simulink library "SimpleTrackedSurveillanceBlock"  (R2018b)
settings: Solver=VariableStepAuto  StartTime=0.0  StopTime=10.0  RelTol=1e-3
undefined symbols (not defined in the file): ac1_ac2_deVar_ft2ps2, ac1_ac2_dhVar_ft2ps2, ac1_ac2_dnVar_ft2ps2, ac1_ac2_east_position_error_ft, ac1_ac2_east_velocity_error_fps, ac1_ac2_eVar_ft2, ac1_ac2_horizontal_position_jitter_stddev_ft, ac1_ac2_horizontal_velocity_jitter_stddev_fps, ac1_ac2_hVar_ft2, ac1_ac2_north_position_error_ft, ac1_ac2_north_velocity_error_fps, ac1_ac2_nVar_ft2, ac1_ac2_seed1, ac1_ac2_seed2, ac1_ac2_seed3, ac1_ac2_seed4, ac1_ac2_seed5, ac1_ac2_seed6, ac1_ac2_vertical_position_error_ft, ac1_ac2_vertical_position_jitter_stddev_ft, ac1_ac2_vertical_velocity_error_fps, ac1_ac2_vertical_velocity_jitter_stddev_fps, ac1dyn_alt0_ft, ac1dyn_lat0_rad, ac1dyn_lon0_rad
libraries: CreateCovDiagMatrix x1
settings Model: Creator=BI28030  LastModifiedBy=BI28030

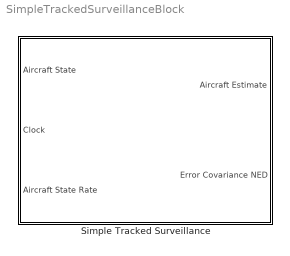
== system SimpleTrackedSurveillanceBlock ==
  Simple Tracked Surveillance : Subsystem  mask(Simple Tracked Surveillance){horizontal_position_jitter_stddev_ft=ac1_ac2_horizontal_position_jitter_stddev_ft, vertical_position_jitter_stddev_ft=ac1_ac2_vertical_position_jitter_stddev_ft, horizontal_velocity_jitter_stddev_fps=ac1_ac2_horizontal_velocity_jitter_stddev_fps, vertical_velocity_jitter_stddev_fps=ac1_ac2_vertical_velocity_jitter_stddev_fps, nVar_ft2=ac1_ac2_nVar_ft2, eVar_ft2=ac1_ac2_eVar_ft2, hVar_ft2=ac1_ac2_hVar_ft2, dnVar_ft2ps2=ac1_ac2_dnVar_ft2ps2, deVar_ft2ps2=ac1_ac2_deVar_ft2ps2, dhVar_ft2ps2=ac1_ac2_dhVar_ft2ps2, seed1=ac1_ac2_seed1, seed2=ac1_ac2_seed2, seed3=ac1_ac2_seed3, seed4=ac1_ac2_seed4, seed5=ac1_ac2_seed5, seed6=ac1_ac2_seed6, east_position_error_ft=ac1_ac2_east_position_error_ft, north_position_error_ft=ac1_ac2_north_position_error_ft, vertical_position_error_ft=ac1_ac2_vertical_position_error_ft, east_velocity_error_fps=ac1_ac2_east_velocity_error_fps, north_velocity_error_fps=ac1_ac2_north_velocity_error_fps, vertical_velocity_error_fps=ac1_ac2_vertical_velocity_error_fps, lat0_rad=ac1dyn_lat0_rad, lon0_rad=ac1dyn_lon0_rad, alt0_ft=ac1dyn_alt0_ft}
      mask prompts: horizontal_position_jitter_stddev_ft "Horizontal Position Jitter Standard Deviation (ft)"; vertical_position_jitter_stddev_ft "Vertical Position Jitter Standard Deviation (ft)"; horizontal_velocity_jitter_stddev_fps "Horizontal Velocity Jitter Standard Deviation (ft/s)"; vertical_velocity_jitter_stddev_fps "Vertical Velocity Jitter Standard Deviation (ft/s)"; nVar_ft2 "Reported Error Covariance: North (ft^2)"; eVar_ft2 "Reported Error Covariance: East (ft^2)"; hVar_ft2 "Reported Error Covariance: Up (ft^2)"; dnVar_ft2ps2 "Reported Error Covariance: North Velocity (ft/s)^2"; deVar_ft2ps2 "Reported Error Covariance: East Velocity (ft/s)^2"; dhVar_ft2ps2 "Reported Error Covariance: Up Velocity (ft/s)^2"; east_position_error_ft "East Position Bias (ft)"; north_position_error_ft "North Position Bias (ft)"; vertical_position_error_ft "Up Position Bias (ft)"; east_velocity_error_fps "East Velocity Bias (ft/s)"; north_velocity_error_fps "North Velocity Bias (ft/s)"; vertical_velocity_error_fps "Up Velocity Bias (ft/s)"; lat0_rad "Latitude of ENU origin (rad)"; lon0_rad "Longitude of ENU origin (rad)"; alt0_ft "Altitude of ENU origin (ft)"
      mask help: Simulates tracked surveillance as constant bias plus white noise
      mask Help:
      | Simulates tracked surveillance as constant bias plus white noise, all Gaussian.
      | 
      | All three components (North, East, Up) are independent.  Velocity and position error are indepdendent.

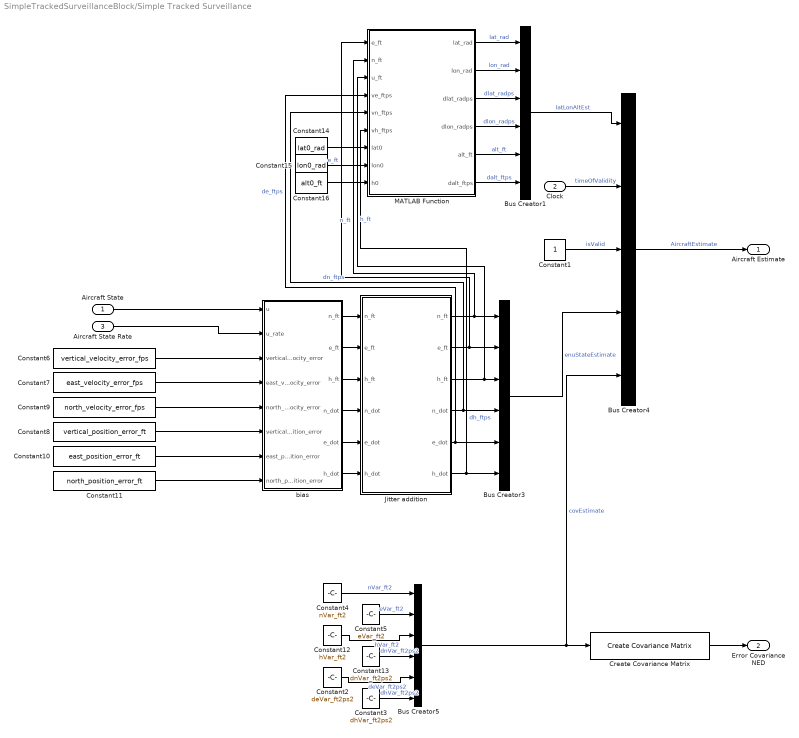
== system SimpleTrackedSurveillanceBlock/Simple Tracked Surveillance ==
  Aircraft State : Inport  OutDataTypeStr=Bus: AircraftState
  Clock : Inport  Port=2
  Aircraft State Rate : Inport  Port=3  OutDataTypeStr=Bus: AircraftStateRate
  Bus Creator1 : BusCreator  Inputs=6  OutDataTypeStr=Bus: LatLonAltMeasurement
  Bus Creator3 : BusCreator  Inputs=6  OutDataTypeStr=Bus: StateEstimate
  Bus Creator4 : BusCreator  Inputs='latLonAltEst','timeOfValidity','isValid','enuStateEstimate','covEstimate'  OutDataTypeStr=Bus: AircraftEstimate  NonVirtualBus=on
  Bus Creator5 : BusCreator  Inputs=6  OutDataTypeStr=Bus: CovarianceEstimate
  Constant1 : Constant  OutDataTypeStr=boolean
  Constant10 : Constant  Value=east_position_error_ft
  Constant11 : Constant  Value=north_position_error_ft
  Constant12 : Constant  Value=hVar_ft2
  Constant13 : Constant  Value=dnVar_ft2ps2
  Constant14 : Constant  Value=lat0_rad  OutDataTypeStr=double
  Constant15 : Constant  Value=lon0_rad  OutDataTypeStr=double
  Constant16 : Constant  Value=alt0_ft  OutDataTypeStr=double
  Constant2 : Constant  Value=deVar_ft2ps2
  Constant3 : Constant  Value=dhVar_ft2ps2
  Constant4 : Constant  Value=nVar_ft2
  Constant5 : Constant  Value=eVar_ft2
  Constant6 : Constant  Value=vertical_velocity_error_fps
  Constant7 : Constant  Value=east_velocity_error_fps
  Constant8 : Constant  Value=vertical_position_error_ft
  Constant9 : Constant  Value=north_velocity_error_fps
  Create Covariance Matrix : CreateCovDiagMatrix/Create Covariance Matrix  SystemSampleTime=-1
  Jitter addition : Subsystem
  MATLAB Function : MATLAB Function  TreatAsAtomicUnit=on
  "bias " : MATLAB Function  TreatAsAtomicUnit=on
  Aircraft Estimate : Outport  OutDataTypeStr=Bus: AircraftEstimate
  Error Covariance NED : Outport  Port=2
  wires:
  Constant11/1 -> "bias "/8(north_position_error)
  Constant10/1 -> "bias "/7(east_position_error)
  Aircraft State Rate/1 -> "bias "/2(u_rate)
  Aircraft State/1 -> "bias "/1(u)
  "bias "/6(h_dot) -> Jitter addition/6("h_dot ")
  "bias "/5(e_dot) -> Jitter addition/5(e_dot)
  "bias "/4(n_dot) -> Jitter addition/4(n_dot)
  "bias "/3(h_ft) -> Jitter addition/3(h_ft)
  "bias "/2(e_ft) -> Jitter addition/2(e_ft)
  "bias "/1(n_ft) -> Jitter addition/1(n_ft)
  Jitter addition/1("n_ft ") -> MATLAB Function/2(n_ft), Bus Creator3/1  "n_ft"
  Jitter addition/2("e_ft ") -> MATLAB Function/1(e_ft), Bus Creator3/2  "e_ft"
  Jitter addition/3("h_ft ") -> MATLAB Function/3(u_ft), Bus Creator3/3  "h_ft"
  Jitter addition/4("n_dot ") -> MATLAB Function/5(vn_ftps), Bus Creator3/4  "dn_ftps"
  Jitter addition/5("e_dot ") -> MATLAB Function/4(ve_ftps), Bus Creator3/5  "de_ftps"
  Jitter addition/6(h_dot) -> MATLAB Function/6(vh_ftps), Bus Creator3/6  "dh_ftps"
  Bus Creator4/1 -> Aircraft Estimate/1  "AircraftEstimate"
  Clock/1 -> Bus Creator4/2  "timeOfValidity"
  Constant1/1 -> Bus Creator4/3  "isValid"
  Bus Creator3/1 -> Bus Creator4/4  "enuStateEstimate"
  Bus Creator5/1 -> Create Covariance Matrix/1, Bus Creator4/5  "covEstimate"
  Constant4/1 -> Bus Creator5/1  "nVar_ft2"
  Constant5/1 -> Bus Creator5/2  "eVar_ft2"
  Constant12/1 -> Bus Creator5/3  "hVar_ft2"
  Constant13/1 -> Bus Creator5/4  "dnVar_ft2ps2"
  Constant2/1 -> Bus Creator5/5  "deVar_ft2ps2"
  Constant3/1 -> Bus Creator5/6  "dhVar_ft2ps2"
  Bus Creator1/1 -> Bus Creator4/1  "latLonAltEst"
  Constant6/1 -> "bias "/3(vertical_velocity_error)
  Constant8/1 -> "bias "/6(vertical_position_error)
  Constant7/1 -> "bias "/4(east_velocity_error)
  Constant9/1 -> "bias "/5(north_velocity_error)
  MATLAB Function/1(lat_rad) -> Bus Creator1/1  "lat_rad"
  MATLAB Function/2(lon_rad) -> Bus Creator1/2  "lon_rad"
  MATLAB Function/3(dlat_radps) -> Bus Creator1/3  "dlat_radps"
  MATLAB Function/4(dlon_radps) -> Bus Creator1/4  "dlon_radps"
  MATLAB Function/5(alt_ft) -> Bus Creator1/5  "alt_ft"
  MATLAB Function/6(dalt_ftps) -> Bus Creator1/6  "dalt_ftps"
  Constant14/1 -> MATLAB Function/7(lat0)
  Constant15/1 -> MATLAB Function/8(lon0)
  Constant16/1 -> MATLAB Function/9(h0)
  Create Covariance Matrix/1 -> Error Covariance NED/1

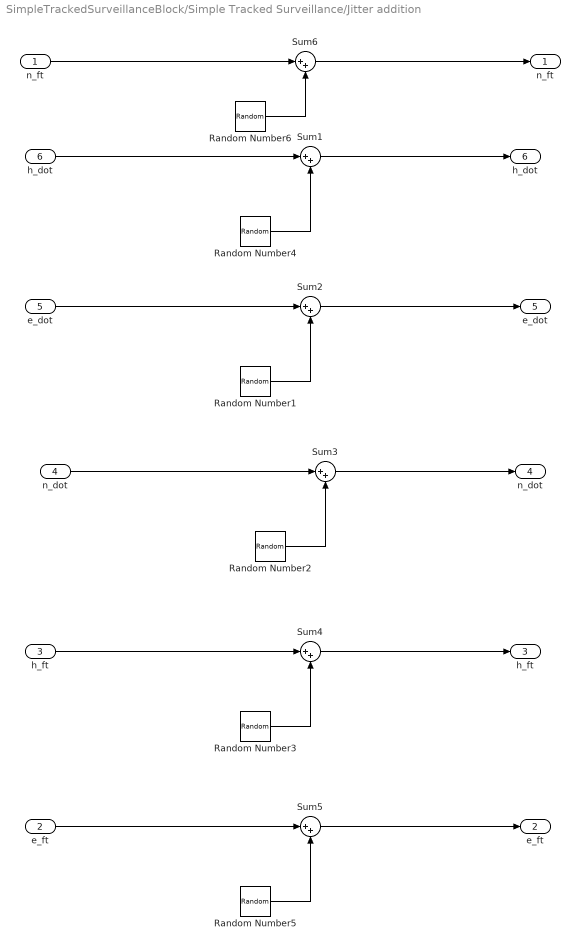
== system SimpleTrackedSurveillanceBlock/Simple Tracked Surveillance/Jitter addition ==
  n_ft : Inport
  e_ft : Inport  Port=2
  h_ft : Inport  Port=3
  n_dot : Inport  Port=4
  e_dot : Inport  Port=5
  "h_dot " : Inport  Port=6
  Random Number1 : RandomNumber  Variance=horizontal_velocity_jitter_stddev_fps.*horizontal_velocity_jitter_stddev_fps  Seed=seed3
  Random Number2 : RandomNumber  Variance=horizontal_velocity_jitter_stddev_fps.*horizontal_velocity_jitter_stddev_fps  Seed=seed4
  Random Number3 : RandomNumber  Variance=vertical_position_jitter_stddev_ft.*vertical_position_jitter_stddev_ft  Seed=seed5
  Random Number4 : RandomNumber  Variance=vertical_velocity_jitter_stddev_fps.*vertical_velocity_jitter_stddev_fps  Seed=seed2
  Random Number5 : RandomNumber  Variance=horizontal_position_jitter_stddev_ft.*horizontal_position_jitter_stddev_ft  Seed=seed6
  Random Number6 : RandomNumber  Variance=horizontal_position_jitter_stddev_ft.*horizontal_position_jitter_stddev_ft  Seed=seed1
  Sum{1..6} (6 alike) : Sum  Inputs=|++
  "n_ft " : Outport  OutDataTypeStr=double
  "e_ft " : Outport  Port=2  OutDataTypeStr=double
  "h_ft " : Outport  Port=3  OutDataTypeStr=double
  "n_dot " : Outport  Port=4  OutDataTypeStr=double
  "e_dot " : Outport  Port=5  OutDataTypeStr=double
  h_dot : Outport  Port=6  OutDataTypeStr=double
  wires:
  "h_dot "/1 -> Sum1/1
  Random Number4/1 -> Sum1/2
  e_dot/1 -> Sum2/1
  Random Number1/1 -> Sum2/2
  n_dot/1 -> Sum3/1
  Random Number2/1 -> Sum3/2
  h_ft/1 -> Sum4/1
  Random Number3/1 -> Sum4/2
  e_ft/1 -> Sum5/1
  Random Number5/1 -> Sum5/2
  n_ft/1 -> Sum6/1
  Random Number6/1 -> Sum6/2
  Sum4/1 -> "h_ft "/1
  Sum5/1 -> "e_ft "/1
  Sum6/1 -> "n_ft "/1
  Sum1/1 -> h_dot/1
  Sum2/1 -> "e_dot "/1
  Sum3/1 -> "n_dot "/1

== matlab function SimpleTrackedSurveillanceBlock/Simple Tracked Surveillance/MATLAB Function ==
  data: e_ft input double size=1; n_ft input double; u_ft input double; ve_ftps input double; vn_ftps input double; vh_ftps input double; lat0 input double; lat_rad output double; lon0 input double; h0 input double; lon_rad output double; dlat_radps output double; dlon_radps output double; alt_ft output double; dalt_ftps output double
function [lat_rad,lon_rad,dlat_radps,dlon_radps,alt_ft,dalt_ftps] = convertToLLA(e_ft,n_ft,u_ft,ve_ftps,vn_ftps,vh_ftps,lat0,lon0,h0)
%#codegen

% WGS-84 ellipsoid constants
a = 2.09256*10^7;          %Semi-major axis (meters)
f = 1.0/298.257223563;  %Flattening
ecc_sq = f*(2.0-f);        %Eccentricity^2


% Ellipsoidal "radius"
er = a./sqrt(1-ecc_sq.*sin(lat0).^2);


% ECEF coordinates
x0 = (er + h0)*cos(lat0)*cos(lon0);
y0 = (er + h0)*cos(lat0)*sin(lon0);
z0 = (er.*(1-ecc_sq) + h0)*sin(lat0);


%% Rotation Matrix
posECEF0 = [x0;y0;z0];
% Compute the local Up unit vector
vHatU = posECEF0;
vHatU(3) = vHatU(3) ./ ((1-f)^2);
vHatU = vHatU ./ norm(vHatU);

% Compute the projection onto the local Up vector
pU = vHatU * vHatU';

% Compute the projection onto the local Tangent plane
pT = eye(size(pU)) - pU;

% Compute the local North unit vector
vHatZ = [0;0;1];
vHatN = pT * vHatZ;
vHatN = vHatN ./ norm(vHatN);

% Compute the local East unit vector
vHatE = cross(vHatN,vHatU);

% Compute ENU rotation matrix
rotMatENU = zeros(3,3);
rotMatENU(:,1) = vHatE;
rotMatENU(:,2) = vHatN;
rotMatENU(:,3) = vHatU;

tPosECEF = rotMatENU*[e_ft;n_ft;u_ft] + [x0;y0;z0];


%% ECEF to LLA
% WGS-84 derived parameters
b = (1-f).*a;                       %Semi-minor axis (meters)
ecc1_sq = (a.^2 - b.^2)./(a.^2);    %First eccentricity squared
ecc2_sq = (a.^2 - b.^2)./(b.^2);    %Second eccentricity squared


% Length of position vector in equatorial plane
rho = sqrt(tPosECEF(1).^2 + tPosECEF(2).^2);

% Auxillary angle
theta = atan( (tPosECEF(3).*a)./(rho.*b) );

lon_rad = atan2(tPosECEF(2),tPosECEF(1));
lat_rad = atan( (tPosECEF(3) + ecc2_sq.*b.*(sin(theta)).^3)./(rho - ecc1_sq.*a.*(cos(theta)).^3) );

ewRadCurv = a./sqrt(1-ecc1_sq.*sin(lat_rad).^2);

alt_ft = (rho./cos(lat_rad)) - ewRadCurv;


%% Velocities - Project 1 sec into future and use to estimate
dalt_ftps = vh_ftps; % Assume about the same


tPosECEF_1sec = rotMatENU*[e_ft+ve_ftps;...
                           n_ft+vn_ftps;...
                           u_ft] + ...
                           [x0;y0;z0];

% Length of position vector in equatorial plane
rho = sqrt(tPosECEF_1sec(1).^2 + tPosECEF_1sec(2).^2);

% Auxillary angle
theta = atan( (tPosECEF_1sec(3).*a)./(rho.*b) );

lon_rad_1sec = atan2(tPosECEF_1sec(2),tPosECEF_1sec(1));
lat_rad_1sec = atan( (tPosECEF_1sec(3) + ecc2_sq.*b.*(sin(theta)).^3)./(rho - ecc1_sq.*a.*(cos(theta)).^3) );

dlat_radps = lat_rad_1sec - lat_rad;
dlon_radps = lon_rad_1sec - lon_rad;
end

== matlab function SimpleTrackedSurveillanceBlock/Simple Tracked Surveillance/bias  ==
  data: n_ft output; e_ft output; h_ft output; n_dot output; e_dot output; u input Bus: AircraftState size=1; u_rate input Bus: AircraftStateRate size=1; h_dot output; vertical_velocity_error input; east_velocity_error input; north_velocity_error input; vertical_position_error input; east_position_error input; north_position_error input
function [ n_ft, e_ft, h_ft, n_dot, e_dot, h_dot ] = fcn(u,u_rate,vertical_velocity_error, east_velocity_error, north_velocity_error, vertical_position_error, east_position_error, north_position_error   )
%#codegen



h_dot = u_rate.hdot_ftps;
e_dot = u_rate.Edot_ftps;
n_dot = u_rate.Ndot_ftps;

h_dot = h_dot + vertical_velocity_error;
e_dot = e_dot + east_velocity_error;
n_dot = n_dot + north_velocity_error;



h_ft  = u.h_ft + vertical_position_error;
e_ft  = u.e_ft + east_position_error;
n_ft  = u.n_ft + north_position_error;
